simulink model "S1_File_didar_KKS_model"  (R2024a)
settings: Solver=ode14x  StartTime=0  StopTime=180  FixedStep=0.001  RelTol=1e-3
settings Model: Creator=Atif Rehman  LastModifiedBy=Hp
settings SolverCC: SolverJacobianMethodControl=FullPerturbation
settings OptimizationCC: ReuseModelBlockBuffer=off
settings RTWCC: GPUComputeCapability=3.5

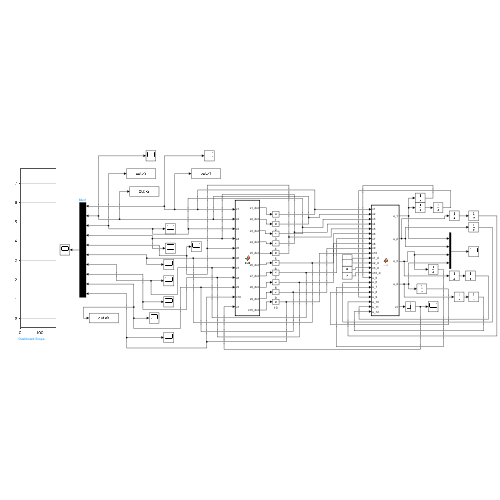
[thumbnail: Simulink's stored preview of the top-level diagram]
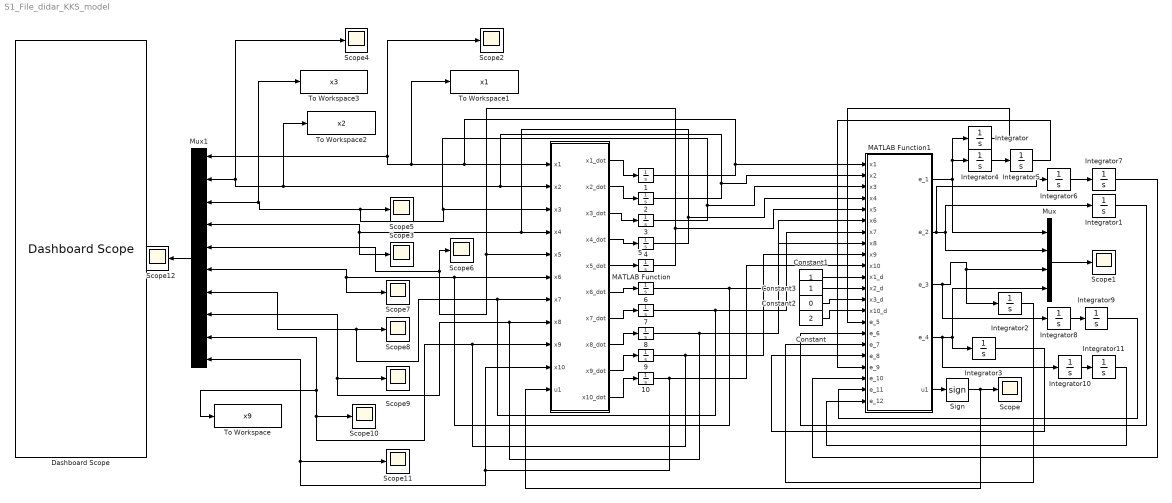
== system S1_File_didar_KKS_model ==
  1 : Integrator  InitialCondition=3.046332648  UpperSaturationLimit=3.046332648  LowerSaturationLimit=0
  10 : Integrator  UpperSaturationLimit=2.0  LowerSaturationLimit=0.2
  2 : Integrator  InitialCondition=4.155524838  UpperSaturationLimit=4.155524838  LowerSaturationLimit=0
  3 : Integrator  InitialCondition=0.0  UpperSaturationLimit=9  LowerSaturationLimit=0
  4 : Integrator  InitialCondition=3.3417*10^(-6)  UpperSaturationLimit=3.34*10^(-6)  LowerSaturationLimit=8.52*10^(-7)
  5 : Integrator  InitialCondition=3.289896258  UpperSaturationLimit=3.289896  LowerSaturationLimit=3
  6 : Integrator  InitialCondition=4.858593207  UpperSaturationLimit=4.8586  LowerSaturationLimit=4
  7 : Integrator  InitialCondition=2.733984514  UpperSaturationLimit=2.73398  LowerSaturationLimit=2.45
  8 : Integrator  UpperSaturationLimit=2  LowerSaturationLimit=0
  9 : Integrator  InitialCondition=3.578358241  UpperSaturationLimit=3.6  LowerSaturationLimit=3.5784
  Constant : Constant  Value=2
  Constant1 : Constant
  Constant2 : Constant  Value=0
  Constant3 : Constant
  Dashboard Scope : DashboardScope
  Integrator{,1..11} (12 alike) : Integrator
  MATLAB Function : MATLAB Function  TreatAsAtomicUnit=on
  MATLAB Function1 : MATLAB Function  TreatAsAtomicUnit=on
  Mux : Mux
  Mux1 : Mux  Inputs=10
  Scope{,1..12} (13 alike) : Scope
  Sign : Signum
  To Workspace : ToWorkspace  VariableName=x9  SampleTime=-1
      settings: Save2DSignal=2-D array (concatenate along first dimension)
  To Workspace1 : ToWorkspace  VariableName=x1  SampleTime=-1
  To Workspace2 : ToWorkspace  VariableName=x2  SampleTime=-1
  To Workspace3 : ToWorkspace  VariableName=x3  SampleTime=-1
  wires:
  Mux/1 -> Scope1/1
  MATLAB Function/1(x1_dot) -> 1/1
  MATLAB Function1/1(e_1) -> Mux/1, Integrator4/1, Integrator/1
  2/1 -> MATLAB Function1/2(x2), MATLAB Function/2(x2), To Workspace2/1, Mux1/2, Scope4/1
  3/1 -> MATLAB Function1/3(x3), MATLAB Function/3(x3), Scope5/1, To Workspace3/1, Mux1/3
  4/1 -> MATLAB Function1/4(x4), Scope3/1, Mux1/4, MATLAB Function/4(x4)
  5/1 -> MATLAB Function1/5(x5), MATLAB Function/5(x5), Scope6/1, Mux1/5
  6/1 -> MATLAB Function1/6(x6), MATLAB Function/6(x6), Mux1/6, Scope7/1
  7/1 -> MATLAB Function1/7(x7), MATLAB Function/7(x7), Scope8/1, Mux1/7
  8/1 -> MATLAB Function1/8(x8), MATLAB Function/8(x8), Mux1/8, Scope9/1
  9/1 -> MATLAB Function1/9(x9), MATLAB Function/9(x9), To Workspace/1, Mux1/9, Scope10/1
  10/1 -> MATLAB Function1/10(x10), MATLAB Function/10(x10), Scope11/1, Mux1/10
  MATLAB Function/2(x2_dot) -> 2/1
  MATLAB Function/3(x3_dot) -> 3/1
  MATLAB Function/4(x4_dot) -> 4/1
  MATLAB Function/5(x5_dot) -> 5/1
  MATLAB Function/6(x6_dot) -> 6/1
  MATLAB Function/7(x7_dot) -> 7/1
  MATLAB Function/8(x8_dot) -> 8/1
  MATLAB Function/9(x9_dot) -> 9/1
  MATLAB Function/10(x10_dot) -> 10/1
  1/1 -> MATLAB Function1/1(x1), MATLAB Function/1(x1), To Workspace1/1, Scope2/1, Mux1/1
  Mux1/1 -> Scope12/1
  Integrator/1 -> MATLAB Function1/15(e_5)
  Integrator1/1 -> MATLAB Function1/16(e_6)
  Integrator3/1 -> MATLAB Function1/18(e_8)
  Integrator2/1 -> MATLAB Function1/17(e_7)
  Integrator4/1 -> Integrator5/1
  Integrator5/1 -> MATLAB Function1/19(e_9)
  Integrator6/1 -> Integrator7/1
  Integrator7/1 -> MATLAB Function1/20(e_10)
  MATLAB Function1/3(e_3) -> Integrator8/1, Integrator2/1, Mux/3
  Integrator8/1 -> Integrator9/1
  Integrator9/1 -> MATLAB Function1/21(e_11)
  MATLAB Function1/4(e_4) -> Integrator10/1, Mux/4, Integrator3/1
  Integrator10/1 -> Integrator11/1
  Integrator11/1 -> MATLAB Function1/22(e_12)
  MATLAB Function1/2(e_2) -> Integrator6/1, Mux/2, Integrator1/1
  MATLAB Function1/5(u1) -> Sign/1
  Sign/1 -> Scope/1, MATLAB Function/11(u1)
  Constant/1 -> MATLAB Function1/14(x10_d)
  Constant1/1 -> MATLAB Function1/11(x1_d)
  Constant2/1 -> MATLAB Function1/13(x3_d)
  Constant3/1 -> MATLAB Function1/12(x2_d)

== matlab function S1_File_didar_KKS_model/MATLAB Function1 ==
  data: x1 input; e_1 output; x2 input; x3 input; x4 input; x5 input; x6 input; x7 input; x8 input; x9 input; x10 input; e_2 output; e_3 output; e_4 output; u1 output; x1_d input; x2_d input; x3_d input; x10_d input; e_5 input; e_6 input; e_7 input; e_8 input; e_9 input; e_10 input; e_11 input; e_12 input
function [e_1,e_2,e_3,e_4,u1] = ctrl(x1,x2,x3,x4,x5,x6,x7,x8,x9,x10,x1_d,x2_d,x3_d,x10_d,e_5,e_6,e_7,e_8,e_9,e_10,e_11,e_12)
%function [e_1,e_2,e_3,e_4,e_5,e_6,e_7,e_8,u1] = ctrl(x1,x2,x3,x4,x5,x6,x7,x8,x9,x10,x1_d,x2_d,x3_d,x10_d)



k_alpha_p=3.4*10^8;
k_alpha_n=1;
k_alpha=0.1;
k_beta=2.8*10^(5);
k_beta_p=0.1;
k_tah_p=8.3*10^7;
k_tah_n=1;
k_sigma_p=8.3*10^(7);
k_gemma_p=2.7*10^(4);
k_mega=0.1;
k_figh_n=0.01;
k_gemma=0.1;
eta_1=0.1;
eta_2=0.1;


%x10=4.155;
%x10=0.83;

x1_dot=-(k_alpha_p)*x1*x2+(k_alpha_n)*x3+k_alpha*x8-k_beta*x1*x4-((eta_1*x1*x10)/(1+x10));
x2_dot=-(k_alpha_p)*x1*x2+(k_alpha_n)*x3-k_gemma*x10*x2;
x3_dot=(k_alpha_p)*x1*x2-(k_alpha_n)*x3-k_mega*x3-((eta_2*x3*x10)/(1+x10));

%c1=0.5;
%c2=1.0;
%c3=1.5;
%c4=2.0;
%k=2;

c1=1e-1;
c2=1e-2;
c3=1e-3;
c4=1e+11;
c5=1e-1;
c6=1e-1;
c7=1e-1;
c8=1e-1;
c9=1e-1;
c10=1e-1;
c11=1e-1;
c12=1e-1;
alpha = 0.5;
beta = 0.5;
k=1e-1;

x1d_dot=0;
x2d_dot=0;
x3d_dot=0;
x4d_dot=0;
x5d_dot=0;
x6d_dot=0;
x7d_dot=0;
x8d_dot=0;
x9d_dot=0;
x10d_dot=0;

e_1=x1-x1_d;
e_2=x2-x2_d;
e_3=x3-x3_d;
e_4=x10-x10_d;

%e_5=int(e_1);
%e_6=int(e_2);
%e_7=int(e_3);
%e_8=int(e_4);

%s= c1*e_1+c2*e_2+c3*e_3+c4*e_4;
%u1=(-1/c4)*(((k)*(abs(s)^(1/2))*sign(s))+c1*(x1_dot-x1d_dot)+c2*(x2_dot-x2d_dot)+c3*(x3_dot-x3d_dot))+x10d_dot+(k_gemma)*x10*x2;


%s= c1*e_1+c2*e_2+c3*e_3+c4*e_4+c5*e_5+c6*e_6+c7*e_7+c8*e_8;
%u1=(-1/c4)*(((k)*(abs(s)^(1/2))*sign(s))+c1*(x1_dot-x1d_dot)+c2*(x2_dot-x2d_dot)+c3*(x3_dot-x3d_dot)+c5*e_1+c6*e_2+c7*e_3+c8*e_4)+x10d_dot+(k_gemma)*x10*x2;

s= c1*e_1+c2*e_2+c3*e_3+c4*e_4+c5*e_5+c6*e_6+c7*e_7+c8*e_8+c9*e_9+c10*e_10+c11*e_11+c12*e_12;
u1=(-1/c4)*(((k)*(abs(s))^(alpha))*sign(s/beta)+c1*(x1_dot-x1d_dot)+c2*(x2_dot-x2d_dot)+c3*(x3_dot-x3d_dot) ...
    +c5*e_1+c6*e_2+c7*e_3+c8*e_4+c9*e_1+c10*e_2+c11*e_3+c12*e_4)+x10d_dot+(k_gemma)*x10*x2;

%u1=0;

== matlab function S1_File_didar_KKS_model/MATLAB Function ==
  data: x1 input; x2 input; x3 input; x4 input; x5 input; x6 input; x7 input; x8 input; x9 input; x10 input; u1 input; x1_dot output; x2_dot output; x3_dot output; x4_dot output; x5_dot output; x6_dot output; x7_dot output; x8_dot output; x9_dot output; x10_dot output
function [x1_dot,x2_dot,x3_dot,x4_dot,x5_dot,x6_dot,x7_dot,x8_dot,x9_dot,x10_dot] = sys(x1,x2,x3,x4,x5,x6,x7,x8,x9,x10,u1)

k_alpha_p=3.4*10^8;
k_alpha_n=1;
k_alpha=0.1;
k_beta=2.8*10^(5);
k_beta_p=0.1;
k_tah_p=8.3*10^7;
k_tah_n=1;
k_sigma_p=8.3*10^(7);
k_gemma_p=2.7*10^(4);
k_mega=0.1;
k_figh_n=0.001;
k_gemma=0.1;
eta_1=0.1;
eta_2=0.1;
%x1=3.0463;
%x2=4.155;
%x3=0.0;
%x4=3.34e-6;
%x5=3.29;
%x6=4.86;
%x7=2.73398;
%x8=0;
%x9=3.6;
%x10=0.85;


% x1 stand for BK, x2 for B2R, x3 for BK:B2R, x4 for TAFIa, x5 for P-KAL,
% x6 for KAL, x7 for HK, x8 for P-KAL:HK, x9 for IL6, and x10 for Icatidant

x1_dot=-(k_alpha_p)*x1*x2+(k_alpha_n)*x3+k_alpha*x8-k_beta*x1*x4-((eta_1*x1*x10)/(1+x10)); 
x2_dot=-(k_alpha_p)*x1*x2+(k_alpha_n)*x3-k_gemma*x10*x2;
x3_dot=(k_alpha_p)*x1*x2-(k_alpha_n)*x3-k_mega*x3-((eta_2*x3*x10)/(1+x10));
x4_dot=-(k_beta_p)*x1*x4;
x5_dot=-(k_gemma_p)*x5*x6-(k_tah_p)*x5*x7+(k_tah_n)*x8;
x6_dot=k_gemma_p*x5*x6-k_sigma_p*x6*x7;
x7_dot=-(k_tah_p)*x5*x7+(k_tah_n)*x8+(k_sigma_p)*x6*x7;
x8_dot=(k_tah_p)*x5*x7-(k_tah_n)*x8-k_alpha*x8;
x9_dot=k_mega*x3-k_figh_n*x9;
x10_dot=-(k_gemma)*x10*x2+u1;
